simulink model "s0102_ref_gen_V1"  (R2021a)
settings: Solver=VariableStepAuto  StartTime=0.0  StopTime=10.0  RelTol=1e-3
values from neighbouring files (symbols this model uses):
  a = [1.5 2.5 5.5 6.5 9.5 10.5 11.5 12.5 13.5 14.5 15.5 16.5 ... (33 elements, 1x33)]    [data_2DLT.mat]    (also in interpolation_test.m = 1)
  b = [0 0.2 0.4 0.6 0.8 1 1.2 1.4 1.6 1.8 2 2.2 ... (142 elements, 1x142)]    [data_2DLT.mat]    (also in interpolation_test.m = 1)
  small_matrix = [0.01 0.01 0.01 0.01 0.0844578553286 0.0367371806961 0.131285467783 0.143327983468 0.191697274148 0.182703464841 0.228217412189 0.220786805561 ... (4686 elements, 33x142)]    [data_2DLT.mat]    (also in interpolation_test.m = zeros(a,b))
settings Model: Creator=ashli  LastModifiedBy=ashli

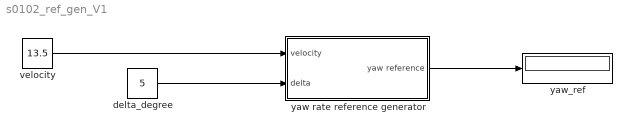
== system s0102_ref_gen_V1 ==
  delta_degree : Constant  Value=5
  velocity : Constant  Value=13.5
  yaw rate reference generator : Subsystem
  yaw_ref : Display
  wires:
  velocity/1 -> yaw rate reference generator/1(velocity)
  delta_degree/1 -> yaw rate reference generator/2(delta)
  yaw rate reference generator/1(yaw reference) -> yaw_ref/1

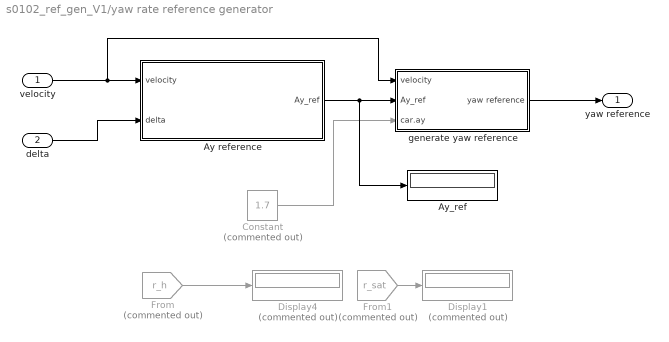
== system s0102_ref_gen_V1/yaw rate reference generator ==
  velocity : Inport
  delta : Inport  Port=2
  Ay reference : Subsystem
  Ay_ref : Display
  Constant : Constant  Commented=on  Value=1.7
  Display1 : Display  Commented=on
  Display4 : Display  Commented=on
  From : From  Commented=on  GotoTag=r_h  TagVisibility=global
  From1 : From  Commented=on  GotoTag=r_sat  TagVisibility=global
  generate yaw reference : Subsystem
  yaw reference : Outport
  wires:
  Constant/1 -> generate yaw reference/3(car.ay)
  From/1 -> Display4/1
  delta/1 -> Ay reference/2(delta)
  generate yaw reference/1(yaw reference) -> yaw reference/1
  velocity/1 -> generate yaw reference/1(velocity), Ay reference/1(velocity)
  Ay reference/1(Ay_ref) -> Ay_ref/1, generate yaw reference/2(Ay_ref)
  From1/1 -> Display1/1

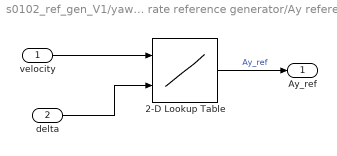
== system s0102_ref_gen_V1/yaw rate reference generator/Ay reference ==
  velocity : Inport
  delta : Inport  Port=2
  2-D Lookup Table : Lookup_n-D  BreakpointsForDimension1=a  BreakpointsForDimension2=b  Table=small_matrix  InternalRulePriority=Speed  RndMeth=Simplest  InputSameDT=on
      settings: InputPortMap=u0,u1
  Ay_ref : Outport
  wires:
  2-D Lookup Table/1 -> Ay_ref/1  "Ay_ref"
  delta/1 -> 2-D Lookup Table/2
  velocity/1 -> 2-D Lookup Table/1

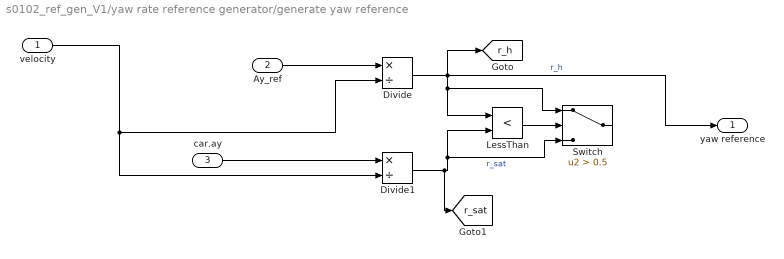
== system s0102_ref_gen_V1/yaw rate reference generator/generate yaw reference ==
  velocity : Inport
  Ay_ref : Inport  Port=2
  car.ay : Inport  Port=3
  Divide : Product  Inputs=*/
  Divide1 : Product  Inputs=*/
  LessThan : RelationalOperator  Operator=<  OutDataTypeStr=boolean  RndMeth=Simplest
  Switch : Switch  Criteria=u2 > Threshold  Threshold=0.5
  yaw reference : Outport
  tag scope: r_h=global, r_sat=global
  wires:
  Divide/1 -> yaw reference/1, [r_h], Switch/1, LessThan/1  "r_h"
  LessThan/1 -> Switch/2
  velocity/1 -> Divide1/2, Divide/2
  car.ay/1 -> Divide1/1
  Divide1/1 -> [r_sat], Switch/3, LessThan/2  "r_sat"
  Ay_ref/1 -> Divide/1
